simulink model "dynamiczny_dyskretny_and_lin"  (R2020a)
settings: Solver=VariableStepAuto  StartTime=0.0  StopTime=100  RelTol=1e-3
values from neighbouring files (symbols this model uses):
  a1 = 0.56    [init_values.m]
  a2 = -0.8    [init_values.m]
  a3 = -0.25    [init_values.m]
  a4 = 0.2    [init_values.m]
  K = 4    [init_values.m]
  T = 1    [test.m]    (also in zad1_10.m; zad1_3.m = 0.1; zad1_9.m)
  T1 = 4    [init_values.m]
  T2 = 10    [init_values.m]
  ulin = sym("ulin")    [test.m]    (also in zad1_10.m; zad1_6.m = -1; zad1_9.m = 1)
settings Model: Creator=jakub  LastModifiedBy=jakub

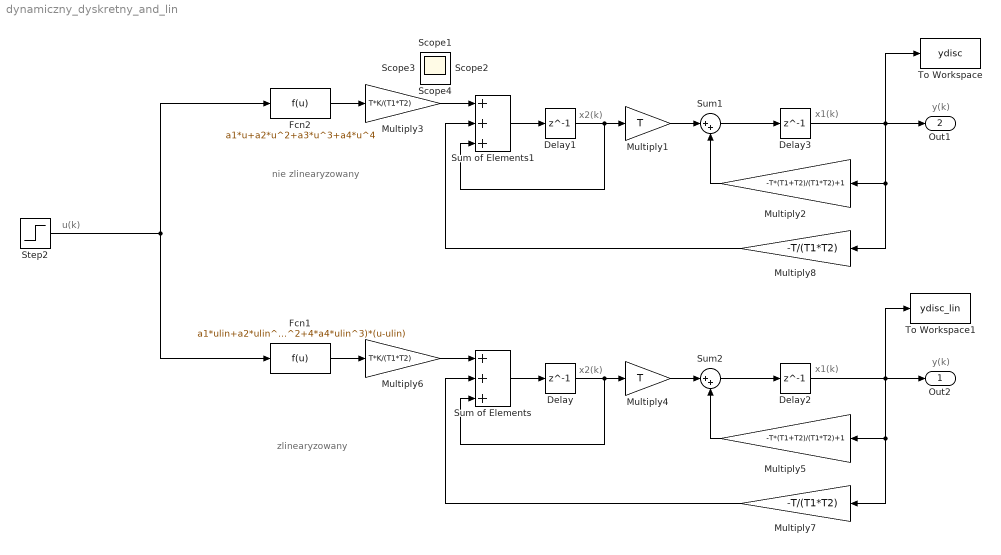
== system dynamiczny_dyskretny_and_lin ==
  note: zlinearyzowany
  note: nie zlinearyzowany
  note: x1(k)
  note: y(k)
  note: x2(k)
  note: x1(k)
  note: y(k)
  note: u(k)
  note: x2(k)
  Delay{,1..3} (4 alike) : Delay  DelayLength=1  InitialCondition=0  SampleTime=T
  Fcn1 : Fcn  Expr=a1*ulin+a2*ulin^2+a3*ulin^3+a4*ulin^4+(a1+2*a2*ulin+3*a3*ulin^2+4*a4*ulin^3)*(u-ulin)
  Fcn2 : Fcn  Expr=a1*u+a2*u^2+a3*u^3+a4*u^4
  Multiply1 : Gain  Gain=T
  Multiply2 : Gain  Gain=-T*(T1+T2)/(T1*T2)+1
  Multiply3 : Gain  Gain=T*K/(T1*T2)
  Multiply4 : Gain  Gain=T
  Multiply5 : Gain  Gain=-T*(T1+T2)/(T1*T2)+1
  Multiply6 : Gain  Gain=T*K/(T1*T2)
  Multiply7 : Gain  Gain=-T/(T1*T2)
  Multiply8 : Gain  Gain=-T/(T1*T2)
  Step2 : Step  Before=-1  SampleTime=0
  Sum of Elements : Sum  Inputs=+++
  Sum of Elements1 : Sum  Inputs=+++
  Sum1 : Sum  Inputs=|++
  Sum2 : Sum  Inputs=|++
  To Workspace : ToWorkspace  VariableName=ydisc  SaveFormat=Structure With Time  SampleTime=T
  To Workspace1 : ToWorkspace  VariableName=ydisc_lin  SaveFormat=Structure With Time  SampleTime=T
  Out2 : Outport
  Out1 : Outport  Port=2
  Scope{1..4} (4 alike) : Scope
  wires:
  Multiply7/1 -> Sum of Elements/2
  Multiply4/1 -> Sum2/1
  Multiply6/1 -> Sum of Elements/1
  Delay2/1 -> To Workspace1/1, Multiply5/1, Multiply7/1, Out2/1
  Fcn1/1 -> Multiply6/1
  Multiply5/1 -> Sum2/2
  Sum of Elements/1 -> Delay/1
  Delay/1 -> Sum of Elements/3, Multiply4/1
  Step2/1 -> Fcn1/1, Fcn2/1
  Sum2/1 -> Delay2/1
  Sum1/1 -> Delay3/1
  Multiply1/1 -> Sum1/1
  Delay3/1 -> To Workspace/1, Out1/1, Multiply2/1, Multiply8/1
  Multiply3/1 -> Sum of Elements1/1
  Multiply2/1 -> Sum1/2
  Multiply8/1 -> Sum of Elements1/2
  Delay1/1 -> Sum of Elements1/3, Multiply1/1
  Sum of Elements1/1 -> Delay1/1
  Fcn2/1 -> Multiply3/1
